simulink model "SzSolo_mic_realtime"  (R2021b)
settings: Solver=FixedStepDiscrete  StartTime=0.0  StopTime=10.0  FixedStep=256/Fs  RelTol=1e-3
PreLoadFcn:
  | Fs = 44100;
  | L = 256;
InitFcn:
  | Fs = 44100;
  | L = 32;
StopFcn:
  | size_ws = size(out.ws);
  | n_rows = size_ws(1);
  | SzEstimado = out.ws(n_rows, :);
libraries: hdlsllib x3, dspsnks4 x2, audiosources x1, simulink x1, sldrtlib x1
settings Model: Creator=Vale Oieni  LastModifiedBy=ValeOieni

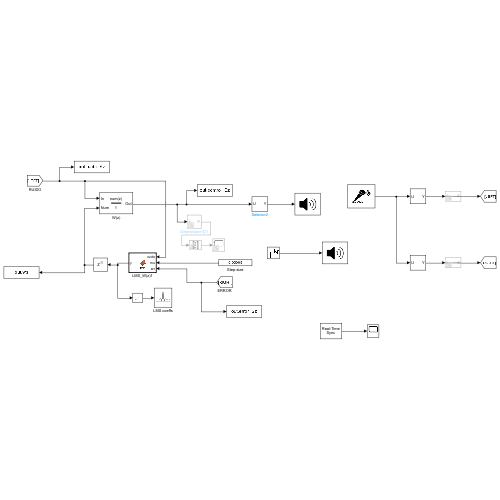
[thumbnail: Simulink's stored preview of the top-level diagram]
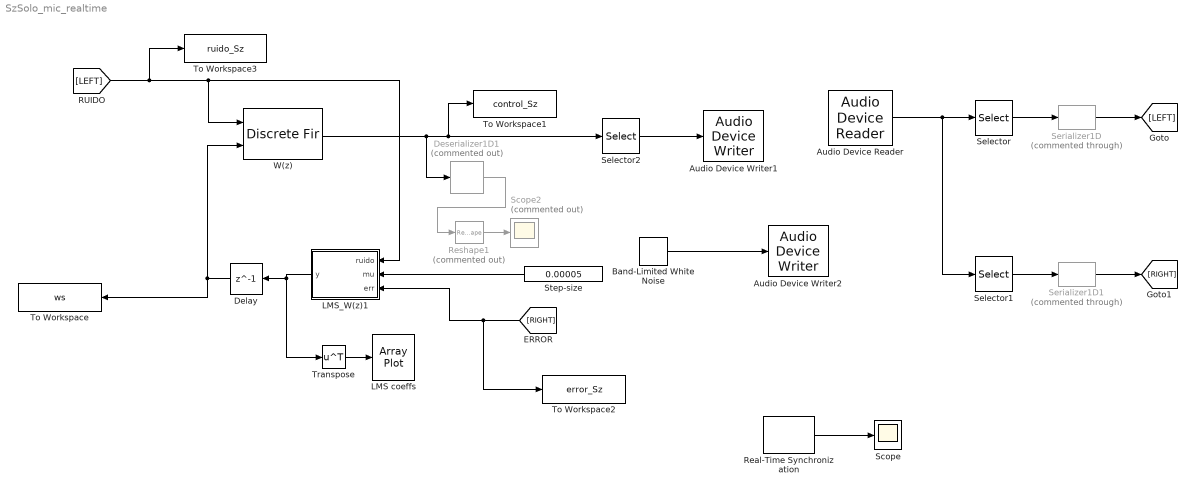
== system SzSolo_mic_realtime ==
  Audio Device Reader : audiosources/Audio Device Reader  Driver=ASIO  Device=ASIO4ALL v2  SampleRate=44100  NumChannels=2  SamplesPerFrame=256  BitDepth=16-bit integer  NumBuffers=10  DefaultInputChannelMapping=on  InputChannelMapping=1:2  OutputNumOverrunSamples=off  OutputDataType=double  DriverIdx=3  DeviceWarnFlag=''
      settings: SourceProductBaseCode=AU
  Audio Device Writer1 : dspsnks4/Audio Device Writer  Driver=ASIO  Device=ASIO4ALL v2  InheritSampleRate=off  SampleRate=44100  BitDepth=16-bit integer  BufferSize=4096  NumBuffers=10  DefaultOutputChannelMapping=on  OutputChannelMapping=1:2  OutputNumUnderrunSamples=off  DriverIdx=3  DeviceWarnFlag=''
  Audio Device Writer2 : dspsnks4/Audio Device Writer  Driver=ASIO  Device=ASIO4ALL v2  InheritSampleRate=off  SampleRate=44100  BitDepth=16-bit integer  BufferSize=4096  NumBuffers=10  DefaultOutputChannelMapping=on  OutputChannelMapping=1:2  OutputNumUnderrunSamples=off  DriverIdx=3  DeviceWarnFlag=''
  Band-Limited White Noise : simulink/Sources/Band-Limited White Noise  Cov=[0.1]  Ts=1/Fs  seed=[23341]
  Delay : Delay  DelayLength=1  InitialCondition=0  InputProcessing=Columns as channels (frame based)
  Deserializer1D1 : hdlsllib/HDL Operations/Deserializer1D  Commented=on  Ratio=256  IdleCycles=0  InitialCondition=0  startIn=off  validIn=off  validOut=off  inputDataDimensions=-1  inputSampleTime=-1  inputSignalType=auto
      settings: SourceProductBaseCode=SL
  LMS coeffs : ArrayPlot  WindowPosition=[301.000000,42.000000,798.000000,828.000000,]  AxesScaling=Manual  YLimits=[-0.624999,0.624999]  ShowLegend=on  DefaultConfigurationName=dsp.scopes.ArrayPlotBlockSpecification
  LMS_W(z)1 : MATLAB Function  TreatAsAtomicUnit=on
  Real-Time Synchronization : sldrtlib/Real-Time Synchronization  SampleTime=256/Fs  MaxMissedTicks=100000  ShowMissedTicks=on  YieldWhenWaiting=off
  Reshape1 : Reshape  Commented=on  OutputDimensionality=Column vector (2-D)  OutputDimensions=[2,1]
  Scope : Scope
  Scope2 : Scope  Commented=on
  Selector : Selector  NumberOfDimensions=2  InputPortWidth=3  IndexOptions=Select all,Index vector (dialog)  Indices=[1 3],1  OutputSizes=1,1
  Selector1 : Selector  NumberOfDimensions=2  InputPortWidth=3  IndexOptions=Select all,Index vector (dialog)  Indices=[1 3],2  OutputSizes=1,1
  Selector2 : Selector  NumberOfDimensions=2  InputPortWidth=3  IndexOptions=Select all,Index vector (dialog)  Indices=[1 3],1  OutputSizes=1,1
  Serializer1D : hdlsllib/HDL Operations/Serializer1D  Commented=through  Ratio=256  IdleCycles=0  validIn=off  startOut=off  validOut=off  inputDataDimensions=-1  inputSampleTime=-1  inputSignalType=auto
      settings: SourceProductBaseCode=SL
  Serializer1D1 : hdlsllib/HDL Operations/Serializer1D  Commented=through  Ratio=256  IdleCycles=0  validIn=off  startOut=off  validOut=off  inputDataDimensions=-1  inputSampleTime=-1  inputSignalType=auto
      settings: SourceProductBaseCode=SL
  Step-size : Constant  Value=0.00005  SampleTime=2048/Fs
  To Workspace : ToWorkspace  VariableName=ws  SampleTime=-1
      settings: Save2DSignal=2-D array (concatenate along first dimension)
  To Workspace1 : ToWorkspace  VariableName=control_Sz  SampleTime=-1
      settings: Save2DSignal=2-D array (concatenate along first dimension)
  To Workspace2 : ToWorkspace  VariableName=error_Sz  SampleTime=-1
      settings: Save2DSignal=2-D array (concatenate along first dimension)
  To Workspace3 : ToWorkspace  VariableName=ruido_Sz  SampleTime=-1
      settings: Save2DSignal=2-D array (concatenate along first dimension)
  Transpose : Math  Operator=transpose  SignedPower=on  SaturateOnIntegerOverflow=on
  W(z) : DiscreteFir  CoefSource=Input port
      settings: InputPortMap=u0,u1
  wires:
  [RIGHT] -> To Workspace2/1, LMS_W(z)1/3(err)
  Delay/1 -> W(z)/2, To Workspace/1
  LMS_W(z)1/1(y) -> Transpose/1, Delay/1
  Transpose/1 -> LMS coeffs/1
  Step-size/1 -> LMS_W(z)1/2(mu)
  Selector1/1 -> Serializer1D1/1
  Audio Device Reader/1 -> Selector1/1, Selector/1
  Selector/1 -> Serializer1D/1
  [LEFT] -> To Workspace3/1, LMS_W(z)1/1(ruido), W(z)/1
  W(z)/1 -> Deserializer1D1/1, To Workspace1/1, Selector2/1
  Serializer1D/1 -> [LEFT]
  Serializer1D1/1 -> [RIGHT]
  Real-Time Synchronization/1 -> Scope/1
  Deserializer1D1/1 -> Reshape1/1
  Reshape1/1 -> Scope2/1
  Selector2/1 -> Audio Device Writer1/1
  Band-Limited White Noise/1 -> Audio Device Writer2/1

== matlab function SzSolo_mic_realtime/LMS_W(z)1 ==
  data: ruido input; mu input; y output; err input
function y = fcn(ruido, mu, err)
    L = 2048;
    %Pesos w_n
    persistent w_n
    if isempty(w_n)
        w_n = zeros(1, L); % inicializa w en cero, largo L
    end
    %Vector de ruido
    persistent x
    if isempty(x)
        x = zeros(1, L); % inicializa x en cero, largo L
    end
    %Vaciado de x
    for i = 1:length(ruido)
        x(2:L) = x(1:L-1);
        x(1) = ruido(i);
        %Actualizacion
        xvar = x;
        w = w_n;
        w = w + mu*err(i)*xvar;   
        w_n = w;
    end
    
    %Asignación a la salida
    y = w;
end
